simulink model "ModeloIdAlfaroLAzoAb"  (R2021a)
settings: Solver=FixedStepAuto  StartTime=0.0  StopTime=200  FixedStep=1e-4  RelTol=1e-3
settings Model: Creator=mluser  LastModifiedBy=Royer

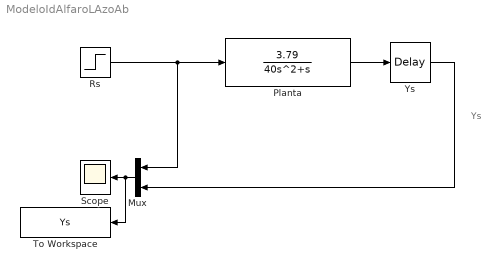
== system ModeloIdAlfaroLAzoAb ==
  note: Ys
  Mux : Mux  Inputs=2
  Planta : TransferFcn  Numerator=[3.79]  Denominator=[40 1 0]  ParameterTunability=Optimized
  Rs : Step  After=10  SampleTime=0
  Scope : Scope
  To Workspace : ToWorkspace  VariableName=Ys  SaveFormat=Timeseries  SampleTime=-1
  Ys : TransportDelay  DelayTime=2
  wires:
  Planta/1 -> Ys/1
  Rs/1 -> Mux/1, Planta/1
  Mux/1 -> To Workspace/1, Scope/1
  Ys/1 -> Mux/2
